simulink model "dpll"  (Simulink 5.0)
settings: Solver=ode45  StartTime=0.0  StopTime=10  RelTol=1e-9  AbsTol=1e-12
values from neighbouring files (symbols this model uses):
  alpha = 2^-24    (= 5.96046447754e-08)    [DPLL_init_2.m]    (also in pt8612_dpll_fpga_init.m = -7; pt8612_dpll_fpga_init_2.m = -5)
  beta = 2^-10    (= 0.0009765625)    [DPLL_init_2.m]    (also in pt8612_dpll_fpga_init.m = 5; pt8612_dpll_fpga_init_2.m = 6)
  C = 680e-9    (= 6.8e-07)    [DPLL_init_2.m]    (also in pt8612_analog_pll_init.m = [1 0]; pt8612_analog_pll_init_2.m = [0 1 0]; pt8612_dpll_fpga_init.m; pt8612_dpll_fpga_init_2.m)
  fvcxo = 148.5e6/1.001    (= 148351648.352)    [DPLL_init_2.m]    (also in pt8612_analog_pll_init.m; pt8612_analog_pll_init_2.m; pt8612_dpll_fpga_init.m; pt8612_dpll_fpga_init_2.m = 148500000)
  Kvcxo = 90e-6    (= 9e-05)    [DPLL_init_2.m]    (also in pt8612_analog_pll_init.m; pt8612_analog_pll_init_2.m; pt8612_dpll_fpga_init.m; pt8612_dpll_fpga_init_2.m)
  Mdac = 3/4    (= 0.75)    [DPLL_init_2.m]    (also in pt8612_dpll_fpga_init.m = 1; pt8612_dpll_fpga_init_2.m = 1)
  Nbits = 16    [DPLL_init_2.m]    (also in pt8612_dpll_fpga_init.m; pt8612_dpll_fpga_init_2.m)
  Ndec1 = 91    [DPLL_init_2.m]    (also in pt8612_analog_pll_init.m; pt8612_analog_pll_init_2.m; pt8612_dpll_fpga_init.m = 364)
  Ndec2 = 500    [DPLL_init_2.m]    (also in pt8612_analog_pll_init.m; pt8612_analog_pll_init_2.m; pt8612_dpll_fpga_init.m = 2000)
  R = 1/(wkneeloop*20)/C    (= 4060.30501089)    [DPLL_init_2.m]    (also in pt8612_dpll_fpga_init.m; pt8612_dpll_fpga_init_2.m = 3900)
  Tpll = 1/fpll    (= 3.37037037037e-06)    [DPLL_init_2.m]    (also in pt8612_dpll_fpga_init.m = 1.34814814815e-05)
  Vcc = 3.3    [DPLL_init_2.m]    (also in pt8612_analog_pll_init.m; pt8612_analog_pll_init_2.m; pt8612_dpll_fpga_init.m = 2.5; pt8612_dpll_fpga_init_2.m = 2.5)
  Vvcxo0 = 1.25    [DPLL_init_2.m]    (also in pt8612_analog_pll_init.m; pt8612_analog_pll_init_2.m; pt8612_dpll_fpga_init.m; pt8612_dpll_fpga_init_2.m)
  Vvcxomax = 2.5    [DPLL_init_2.m]    (also in pt8612_analog_pll_init.m; pt8612_analog_pll_init_2.m; pt8612_dpll_fpga_init.m; pt8612_dpll_fpga_init_2.m)
  Vvcxomin = 0    [DPLL_init_2.m]    (also in pt8612_analog_pll_init.m; pt8612_analog_pll_init_2.m; pt8612_dpll_fpga_init.m; pt8612_dpll_fpga_init_2.m)
libraries: simulink x3
settings Model: LastModifiedBy=thh

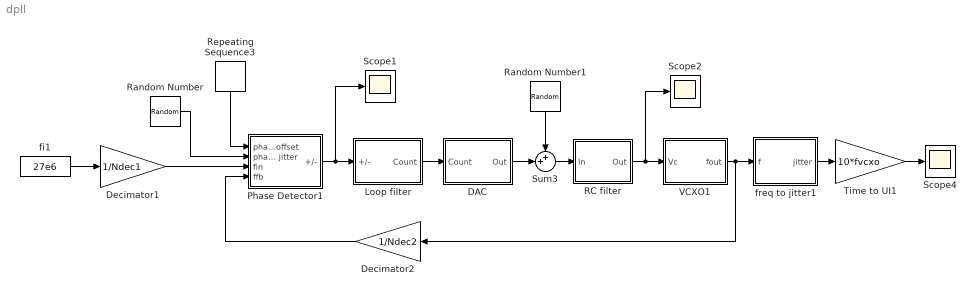
== system dpll ==
  DAC : Subsystem
  Decimator1 : Gain  Gain=1/Ndec1  SaturateOnIntegerOverflow=on
  Decimator2 : Gain  Orientation=left  Gain=1/Ndec2  SaturateOnIntegerOverflow=on
  Loop filter : Subsystem
  Phase Detector1 : Subsystem
  RC filter : Subsystem
  Random Number : RandomNumber  Variance=0.05  SampleTime=Tpll
  Random Number1 : RandomNumber  Orientation=down  Variance=0.1e-3  SampleTime=Tpll
  Repeating Sequence3 : simulink/Sources/Repeating Sequence  Orientation=down  rep_seq_t=[0 0.5 0.5 1]*5  rep_seq_y=[0 0 1 1]*5
  Scope1 : Scope
      settings: TimeRange=10  YMin=-30  YMax=180
  Scope2 : Scope
      settings: TimeRange=10  YMin=1.2496  YMax=1.2511  SaveName=ScopeData3
  Scope4 : Scope
      settings: TimeRange=10  YMin=-10  YMax=55  SaveName=ScopeData2
  Sum3 : Sum  Inputs=++|  SaturateOnIntegerOverflow=on
  Time to UI1 : Gain  Gain=10*fvcxo  SaturateOnIntegerOverflow=on
  VCXO1 : Subsystem
  fi1 : Constant  Value=27e6
  freq to jitter1 : Subsystem
  wires:
  freq to jitter1/1(jitter) -> Time to UI1/1
  Time to UI1/1 -> Scope4/1
  VCXO1/1(fout) -> freq to jitter1/1(f), Decimator2/1
  Decimator2/1 -> Phase Detector1/4(ffb)
  Phase Detector1/1(+/-) -> Loop filter/1(+/-), Scope1/1
  Decimator1/1 -> Phase Detector1/3(fin)
  fi1/1 -> Decimator1/1
  Loop filter/1(Count) -> DAC/1(Count)
  RC filter/1(Out) -> VCXO1/1(Vc), Scope2/1
  Repeating Sequence3/1 -> Phase Detector1/1(phase offset)
  Random Number/1 -> Phase Detector1/2(phase jitter)
  DAC/1(Out) -> Sum3/2
  Sum3/1 -> RC filter/1(In)
  Random Number1/1 -> Sum3/1

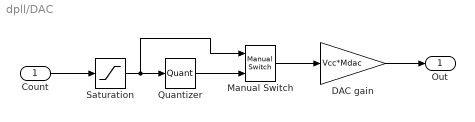
== system dpll/DAC ==
  Count : Inport
  DAC gain : Gain  Gain=Vcc*Mdac  SaturateOnIntegerOverflow=on
  Manual Switch : simulink/Signal Routing/Manual Switch  sw=0  action=0
  Quantizer : Quantizer  QuantizationInterval=2^-Nbits
  Saturation : Saturate  UpperLimit=1  LowerLimit=0
  Out : Outport
  wires:
  DAC gain/1 -> Out/1
  Count/1 -> Saturation/1
  Saturation/1 -> Quantizer/1, Manual Switch/1
  Manual Switch/1 -> DAC gain/1
  Quantizer/1 -> Manual Switch/2

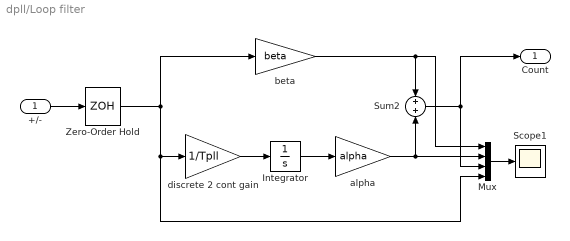
== system dpll/Loop filter ==
  +/- : Inport
  Integrator : Integrator
  Mux : Mux
  Scope1 : Scope
      settings: TimeRange=10  YMin=-0.5  YMax=6.5  SaveName=ScopeData5
  Sum2 : Sum  SaturateOnIntegerOverflow=on
  Zero-Order Hold : ZeroOrderHold  SampleTime=Tpll
  alpha : Gain  Gain=alpha  SaturateOnIntegerOverflow=on
  beta : Gain  Gain=beta  SaturateOnIntegerOverflow=on
  discrete 2 cont gain : Gain  Gain=1/Tpll  SaturateOnIntegerOverflow=on
  Count : Outport
  wires:
  +/-/1 -> Zero-Order Hold/1
  Sum2/1 -> Count/1, Mux/3
  beta/1 -> Sum2/1, Mux/1
  alpha/1 -> Sum2/2, Mux/2
  Mux/1 -> Scope1/1
  Integrator/1 -> alpha/1
  discrete 2 cont gain/1 -> Integrator/1
  Zero-Order Hold/1 -> beta/1, discrete 2 cont gain/1, Mux/4

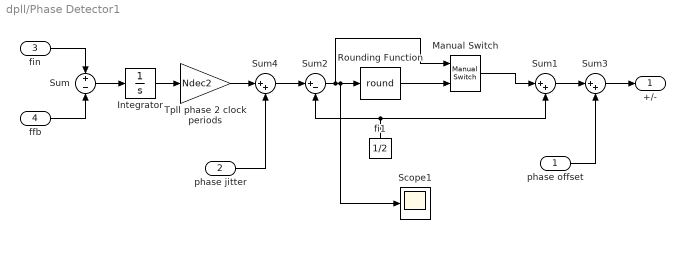
== system dpll/Phase Detector1 ==
  phase offset : Inport
  phase jitter : Inport  Port=2
  fin : Inport  Port=3
  ffb : Inport  Port=4
  Integrator : Integrator
  Manual Switch : simulink/Signal Routing/Manual Switch  sw=0  action=0
  Rounding Function : Rounding  Operator=round
  Scope1 : Scope
      settings: TimeRange=10  YMin=-0.5  YMax=6.5
  Sum : Sum  Inputs=+-  SaturateOnIntegerOverflow=on
  Sum1 : Sum  Inputs=|++  SaturateOnIntegerOverflow=on
  Sum2 : Sum  Inputs=|+-  SaturateOnIntegerOverflow=on
  Sum3 : Sum  Inputs=|++  SaturateOnIntegerOverflow=on
  Sum4 : Sum  Inputs=|++  SaturateOnIntegerOverflow=on
  Tpll phase 2 clock periods : Gain  Gain=Ndec2  SaturateOnIntegerOverflow=on
  fi1 : Constant  Orientation=up  Value=1/2
  +/- : Outport
  wires:
  ffb/1 -> Sum/2
  fin/1 -> Sum/1
  Sum/1 -> Integrator/1
  Integrator/1 -> Tpll phase 2 clock periods/1
  fi1/1 -> Sum1/2, Sum2/2
  Sum2/1 -> Manual Switch/1, Rounding Function/1, Scope1/1
  phase offset/1 -> Sum3/2
  Sum3/1 -> +/-/1
  Sum1/1 -> Sum3/1
  Manual Switch/1 -> Sum1/1
  Rounding Function/1 -> Manual Switch/2
  phase jitter/1 -> Sum4/2
  Sum4/1 -> Sum2/1
  Tpll phase 2 clock periods/1 -> Sum4/1

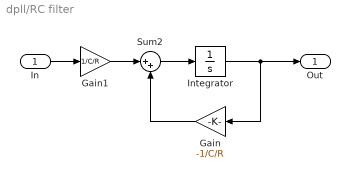
== system dpll/RC filter ==
  In : Inport
  Gain : Gain  Orientation=left  Gain=-1/C/R  SaturateOnIntegerOverflow=on
  Gain1 : Gain  Gain=1/C/R  SaturateOnIntegerOverflow=on
  Integrator : Integrator  InitialCondition=Vvcxo0
  Sum2 : Sum  Inputs=|++  SaturateOnIntegerOverflow=on
  Out : Outport
  wires:
  In/1 -> Gain1/1
  Integrator/1 -> Out/1, Gain/1
  Sum2/1 -> Integrator/1
  Gain/1 -> Sum2/2
  Gain1/1 -> Sum2/1

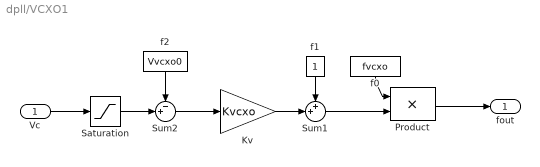
== system dpll/VCXO1 ==
  Vc : Inport
  Kv : Gain  Gain=Kvcxo  SaturateOnIntegerOverflow=on
  Product : Product  SaturateOnIntegerOverflow=on
  Saturation : Saturate  UpperLimit=Vvcxomax  LowerLimit=Vvcxomin
  Sum1 : Sum  Inputs=++|  SaturateOnIntegerOverflow=on
  Sum2 : Sum  Inputs=-+|  SaturateOnIntegerOverflow=on
  f0 : Constant  Orientation=down  Value=fvcxo
  f1 : Constant  Orientation=down
  f2 : Constant  Orientation=down  Value=Vvcxo0
  fout : Outport
  wires:
  f2/1 -> Sum2/1
  Vc/1 -> Saturation/1
  Sum2/1 -> Kv/1
  Product/1 -> fout/1
  Kv/1 -> Sum1/2
  Sum1/1 -> Product/2
  f1/1 -> Sum1/1
  f0/1 -> Product/1
  Saturation/1 -> Sum2/2

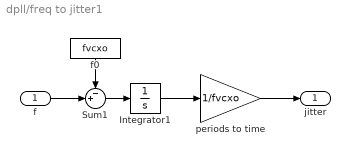
== system dpll/freq to jitter1 ==
  f : Inport
  Integrator1 : Integrator
  Sum1 : Sum  Inputs=-+|  SaturateOnIntegerOverflow=on
  f0 : Constant  Orientation=down  Value=fvcxo
  periods to time : Gain  Gain=1/fvcxo  SaturateOnIntegerOverflow=on
  jitter : Outport
  wires:
  periods to time/1 -> jitter/1
  f/1 -> Sum1/2
  f0/1 -> Sum1/1
  Sum1/1 -> Integrator1/1
  Integrator1/1 -> periods to time/1
